simulink model "Q1sim"  (R2021b)
settings: Solver=VariableStepAuto  StartTime=0.0  StopTime=10.0  RelTol=1e-3
values from neighbouring files (symbols this model uses):
  K_fast = place(A,B,p_fast)    [Q1.m]    (also in Q3.m)
  K_slow = place(A,B,p_slow)    [Q1.m]    (also in Q3.m)
settings Model: Creator=Siavash  LastModifiedBy=Siavash
settings SolverCC: AlgebraicLoopSolver=TrustRegion
settings DataIOCC: ReturnWorkspaceOutputs=off
settings DebuggingCC: SFMachineParentedDataDiag=warning  ArithmeticOperatorsInVariantConditions=warning
settings SFSimCC: SimUseLocalCustomCode=off  CustomCodeUndefinedFunction=UseInterfaceOnly
settings RTWCC: RTWUseLocalCustomCode=off

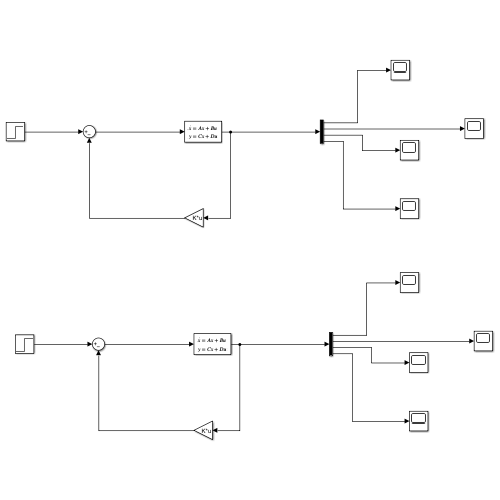
[thumbnail: Simulink's stored preview of the top-level diagram]
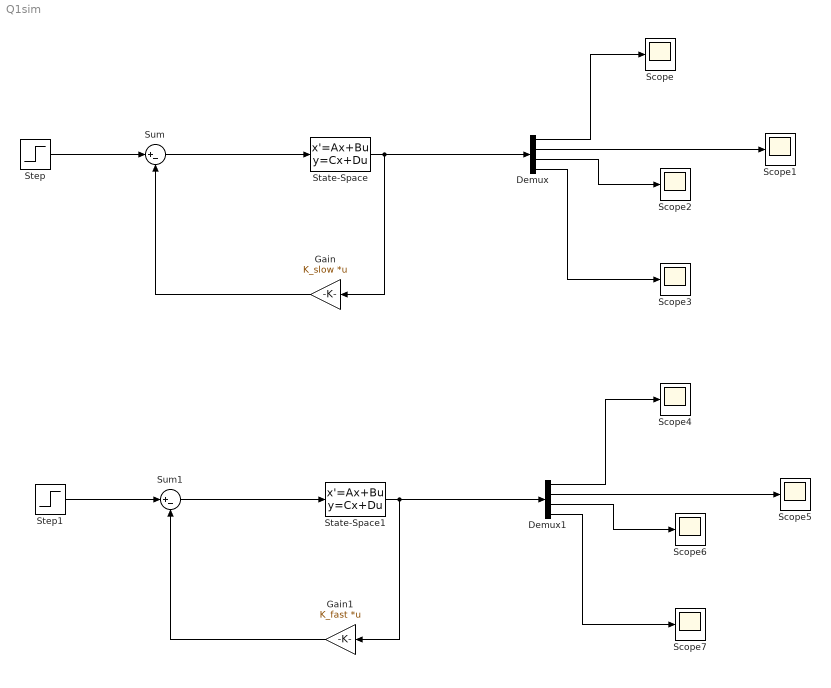
== system Q1sim ==
  Demux : Demux
  Demux1 : Demux
  Gain : Gain  Gain=K_slow  Multiplication=Matrix(K*u)
  Gain1 : Gain  Gain=K_fast  Multiplication=Matrix(K*u)
  Scope{,1..7} (8 alike) : Scope
  State-Space : StateSpace  A=[0 1 0 0 ;0 -2.2626 -0.3962 -0.0082; 0 0 0 1;0 3.5649 16.0655 -0.3324]  B=[0; 0.2263; 0; -0.3565]  C=eye(4,4)  D=[0;0;0;0]  InitialCondition=0
  State-Space1 : StateSpace  A=[0 1 0 0 ;0 -2.2626 -0.3962 -0.0082; 0 0 0 1;0 3.5649 16.0655 -0.3324]  B=[0; 0.2263; 0; -0.3565]  C=eye(4,4)  D=[0;0;0;0]  InitialCondition=0
  Step : Step  Time=0  SampleTime=0
  Step1 : Step  Time=0  SampleTime=0
  Sum : Sum  Inputs=|+-
  Sum1 : Sum  Inputs=|+-
  wires:
  State-Space/1 -> Demux/1, Gain/1
  Demux/1 -> Scope/1
  Demux/2 -> Scope1/1
  Demux/3 -> Scope2/1
  Demux/4 -> Scope3/1
  Sum/1 -> State-Space/1
  Gain/1 -> Sum/2
  Step/1 -> Sum/1
  Demux1/3 -> Scope6/1
  Demux1/2 -> Scope5/1
  Sum1/1 -> State-Space1/1
  Demux1/1 -> Scope4/1
  Gain1/1 -> Sum1/2
  State-Space1/1 -> Demux1/1, Gain1/1
  Demux1/4 -> Scope7/1
  Step1/1 -> Sum1/1
